simulink model "svpwm"  (R2018a)
settings: Solver=VariableStepAuto  StartTime=0.0  StopTime=5  MaxStep=1e-7  RelTol=1e-3
libraries: simulink x1
settings Model: Creator=R-YDL  LastModifiedBy=R-YDL

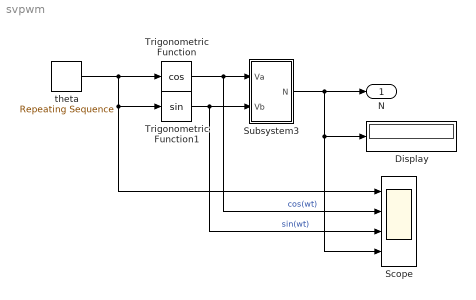
== system svpwm ==
  Display : Display
  Scope : Scope  NumInputPorts=4
  Subsystem3 : Subsystem
  Trigonometric Function : Trigonometry  Operator=cos
  Trigonometric Function1 : Trigonometry
  theta : simulink/Sources/Repeating Sequence  rep_seq_t=[0 1]  rep_seq_y=[0 2]*pi
  "N " : Outport
  wires:
  theta/1 -> Trigonometric Function/1, Trigonometric Function1/1, Scope/1
  Trigonometric Function/1 -> Scope/2, Subsystem3/1(Va)  "cos(wt)"
  Trigonometric Function1/1 -> Subsystem3/2("Vb "), Scope/3  "sin(wt)"
  Subsystem3/1("N ") -> "N "/1, Display/1, Scope/4

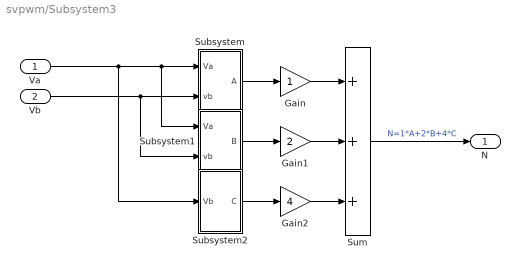
== system svpwm/Subsystem3 ==
  Va : Inport
  "Vb " : Inport  Port=2
  Gain : Gain
  Gain1 : Gain  Gain=2
  Gain2 : Gain  Gain=4
  Subsystem : Subsystem
  Subsystem1 : Subsystem
  Subsystem2 : Subsystem
  Sum : Sum  Inputs=+++
  "N " : Outport
  wires:
  Sum/1 -> "N "/1  "N=1*A+2*B+4*C"
  Va/1 -> Subsystem2/1("Vb "), Subsystem1/1(Va), Subsystem/1(Va)
  Subsystem2/1(C) -> Gain2/1
  "Vb "/1 -> Subsystem1/2("vb "), Subsystem/2("vb ")
  Subsystem1/1(B) -> Gain1/1
  Gain/1 -> Sum/1
  Subsystem/1(A) -> Gain/1
  Gain1/1 -> Sum/2
  Gain2/1 -> Sum/3

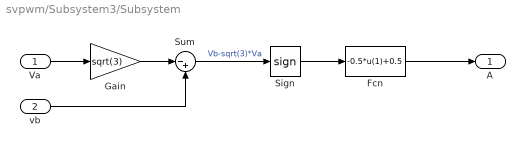
== system svpwm/Subsystem3/Subsystem ==
  Va : Inport
  "vb " : Inport  Port=2
  Fcn : Fcn  Expr=-0.5*u(1)+0.5
  Gain : Gain  Gain=sqrt(3)
  Sign : Signum
  Sum : Sum  Inputs=|-+
  A : Outport
  wires:
  Va/1 -> Gain/1
  "vb "/1 -> Sum/2
  Gain/1 -> Sum/1
  Fcn/1 -> A/1
  Sum/1 -> Sign/1  "Vb-sqrt(3)*Va"
  Sign/1 -> Fcn/1

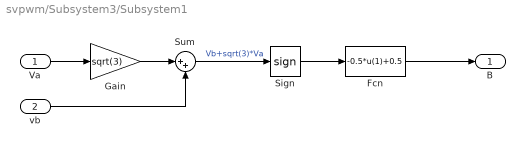
== system svpwm/Subsystem3/Subsystem1 ==
  Va : Inport
  "vb " : Inport  Port=2
  Fcn : Fcn  Expr=-0.5*u(1)+0.5
  Gain : Gain  Gain=sqrt(3)
  Sign : Signum
  Sum : Sum  Inputs=|++
  B : Outport
  wires:
  Va/1 -> Gain/1
  "vb "/1 -> Sum/2
  Gain/1 -> Sum/1
  Fcn/1 -> B/1
  Sum/1 -> Sign/1  "Vb+sqrt(3)*Va"
  Sign/1 -> Fcn/1

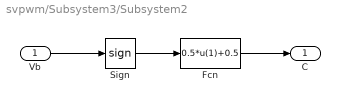
== system svpwm/Subsystem3/Subsystem2 ==
  "Vb " : Inport
  Fcn : Fcn  Expr=0.5*u(1)+0.5
  Sign : Signum
  C : Outport
  wires:
  Fcn/1 -> C/1
  Sign/1 -> Fcn/1
  "Vb "/1 -> Sign/1
